simulink model "modelo_asm1_v2"  (R2024a)
settings: Solver=VariableStepAuto  StartTime=0.0  StopTime=28  RelTol=1e-3  AbsTol=Auto  EnableMultiTasking=on
settings Model: Creator=romeroj  LastModifiedBy=ktb21
settings DataIOCC: ExternalInput=dat.data  SaveFormat=Array  SignalLoggingSaveFormat=ModelDataLogs  ReturnWorkspaceOutputs=off
settings OptimizationCC: BooleanDataType=off  ExpressionDepthLimit=2147483647  InitFltsAndDblsToZero=on  LifeSpan=inf
settings DebuggingCC: SaveWithParameterizedLinksMsg=none  UnderspecifiedInitializationDetection=Classic  MergeDetectMultiDrivingBlocksExec=none  SignalResolutionControl=TryResolveAllWithWarning  MultiTaskDSMMsg=warning  MultiTaskCondExecSysMsg=none  FcnCallInpInsideContextMsg=warning  UnconnectedInputMsg=warning  UnconnectedOutputMsg=warning  UnconnectedLineMsg=warning  StateNameClashWarn=warning  SFUnexpectedBacktrackingDiag=warning  SFNoUnconditionalDefaultTransitionDiag=warning  ArithmeticOperatorsInVariantConditions=warning
settings HardwareCC: ProdBitPerPointer=32  ProdBitPerSizeT=32  ProdBitPerPtrDiffT=32  ProdLargestAtomicFloat=None  ProdIntDivRoundTo=Undefined  ProdEndianess=Unspecified  ProdWordSize=32  ProdHWDeviceType=32-bit Generic  TargetUnknown=on
settings ModelReferenceCC: EnableRefExpFcnMdlSchedulingChecks=on  PropagateSignalLabelsOutOfModel=off
settings SFSimCC: SimUseLocalCustomCode=off  SimParseCustomCode=off  CustomCodeUndefinedFunction=UseInterfaceOnly
settings RTWCC: RTWUseLocalCustomCode=off  GPUComputeCapability=3.5
settings CodeAppCC: StateflowObjectComments=on
settings GRTTargetCC: TargetFcnLib=ansi_tfl_tmw.mat  TargetLangStandard=C89/C90 (ANSI)  CombineOutputUpdateFcns=off  GRTInterface=on
settings ConfigComp: CovMetricSettings=dw  CovSaveCumulativeToWorkspaceVar=on  CovSaveSingleToWorkspaceVar=on  CovExternalEMLEnable=off

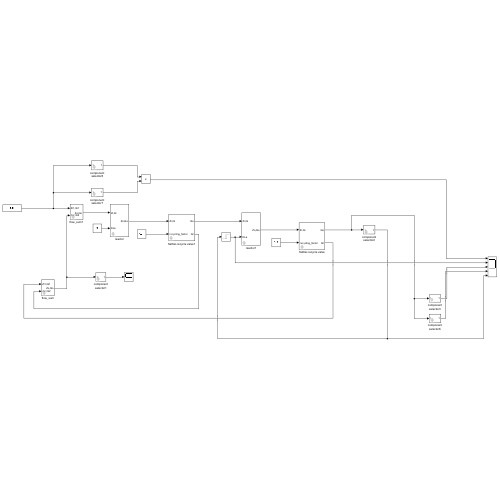
[thumbnail: Simulink's stored preview of the top-level diagram]
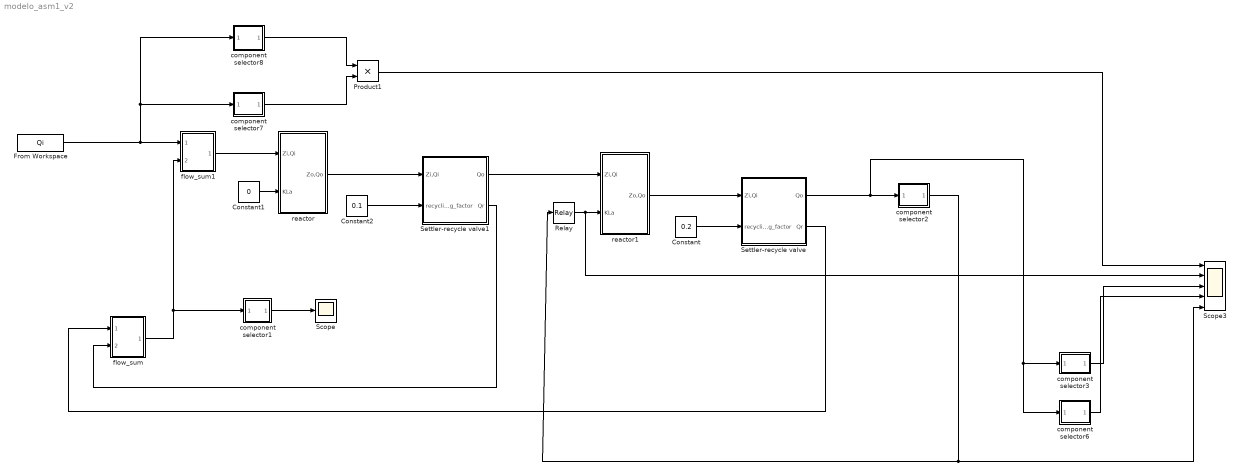
== system modelo_asm1_v2 ==
  Constant : Constant  Value=0.2
  Constant1 : Constant  Value=0
  Constant2 : Constant  Value=0.1
  From Workspace : FromWorkspace  VariableName=Qi  SampleTime=2/1440  ZeroCross=off  OutputAfterFinalValue=Holding final value
  Product1 : Product  RndMeth=Zero
  Relay : Relay  OnSwitchValue=5.4  OffSwitchValue=3  OnOutputValue=40
  Scope : Scope
  Scope3 : Scope  NumInputPorts=5
  Settler-recycle valve : Subsystem  mask{nXi=4, nXs=4, nXbh=4, nXba=4, nXp=4}
      mask prompts: nXi "Xi"; nXs "Xs"; nXbh "Xbh"; nXba "Xba"; nXp "Xp"
      mask DialogControl ParameterTabVar0 Prompt: Settler coefficients
  Settler-recycle valve1 : Subsystem  mask{nXi=0, nXs=0, nXbh=0, nXba=0, nXp=0}
      mask prompts: nXi "Xi"; nXs "Xs"; nXbh "Xbh"; nXba "Xba"; nXp "Xp"
      mask DialogControl ParameterTabVar0 Prompt: Settler coefficients
  component selector1 : Subsystem  mask(Component selection){si=off, ss=off, xi=off, xs=off, xbh=off, xba=off, xp=off, so=off, sno=off, snh=off, snd=off, xnd=off, salk=off, Q=on}
      mask prompts: si "Si: Soluble inert organic matter"; ss "Ss: Readily biodegradable substrate"; xi "Xi: Particulate inert organic matter"; xs "Xs: Slowly biodegradable substrate"; xbh "Xbh: Active heterotrophic biomass"; xba "Xba: Active autotrophic biomass"; xp "Xp: Particulate products arising from biomass decay"; so "So: Oxygen"; sno "Sno: Nitrate and nitrite nitrogen"; snh "Snh: NH 4+ + NH 3 nitrogen"; snd "Snd: Soluble biodegradable organic nitrogen"; xnd "Xnd: Particulate biodegradable organic nitrogen"; salk "Salk: Alkalinity"; Q "Q: Flowrate"
      mask help: Select the components to appear in the output vector of this block.
      mask init:
      | if si
      |     indexx=[1];
      | else
      |     indexx=[];
      | end
      | if ss
      |     indexx=[indexx 2];
      | end
      | if xi
      |     indexx=[indexx 3];
      | end
      | if xs
      |     indexx=[indexx 4];
      | end
      | if xbh
      |     indexx=[indexx 5];
      | end
      | if xba
      |     indexx=[indexx 6];
      | end
      | if xp
      |     indexx=[indexx 7];
      | end
      | if so
      |     indexx=[indexx 8];
      | end
      | if sno
      |     indexx=[indexx 9];
      | end
      | if snh
      |     indexx=[indexx 10];
      | end
      | if snd
      |     indexx=[indexx 11];
      | end
      | if xnd
      |     indexx=[indexx 12];
      | end
      | if salk
      |     indexx=[indexx 13]
      | end
      | if Q
      |     indexx=[indexx 14]
      | end
  component selector2 : Subsystem  mask(Component selection){si=off, ss=off, xi=off, xs=off, xbh=off, xba=off, xp=off, so=off, sno=off, snh=on, snd=off, xnd=off, salk=off, Q=off}
      mask prompts: si "Si: Soluble inert organic matter"; ss "Ss: Readily biodegradable substrate"; xi "Xi: Particulate inert organic matter"; xs "Xs: Slowly biodegradable substrate"; xbh "Xbh: Active heterotrophic biomass"; xba "Xba: Active autotrophic biomass"; xp "Xp: Particulate products arising from biomass decay"; so "So: Oxygen"; sno "Sno: Nitrate and nitrite nitrogen"; snh "Snh: NH 4+ + NH 3 nitrogen"; snd "Snd: Soluble biodegradable organic nitrogen"; xnd "Xnd: Particulate biodegradable organic nitrogen"; salk "Salk: Alkalinity"; Q "Q: Flowrate"
      mask help: Select the components to appear in the output vector of this block.
      mask init: same as modelo_asm1_v2/component selector1
  component selector3 : Subsystem  mask(Component selection){si=off, ss=off, xi=off, xs=off, xbh=off, xba=off, xp=off, so=on, sno=off, snh=off, snd=off, xnd=off, salk=off, Q=off}
      mask prompts: si "Si: Soluble inert organic matter"; ss "Ss: Readily biodegradable substrate"; xi "Xi: Particulate inert organic matter"; xs "Xs: Slowly biodegradable substrate"; xbh "Xbh: Active heterotrophic biomass"; xba "Xba: Active autotrophic biomass"; xp "Xp: Particulate products arising from biomass decay"; so "So: Oxygen"; sno "Sno: Nitrate and nitrite nitrogen"; snh "Snh: NH 4+ + NH 3 nitrogen"; snd "Snd: Soluble biodegradable organic nitrogen"; xnd "Xnd: Particulate biodegradable organic nitrogen"; salk "Salk: Alkalinity"; Q "Q: Flowrate"
      mask help: Select the components to appear in the output vector of this block.
      mask init: same as modelo_asm1_v2/component selector1
  component selector6 : Subsystem  mask(Component selection){si=off, ss=off, xi=on, xs=off, xbh=off, xba=off, xp=off, so=off, sno=off, snh=off, snd=off, xnd=off, salk=off, Q=off}
      mask prompts: si "Si: Soluble inert organic matter"; ss "Ss: Readily biodegradable substrate"; xi "Xi: Particulate inert organic matter"; xs "Xs: Slowly biodegradable substrate"; xbh "Xbh: Active heterotrophic biomass"; xba "Xba: Active autotrophic biomass"; xp "Xp: Particulate products arising from biomass decay"; so "So: Oxygen"; sno "Sno: Nitrate and nitrite nitrogen"; snh "Snh: NH 4+ + NH 3 nitrogen"; snd "Snd: Soluble biodegradable organic nitrogen"; xnd "Xnd: Particulate biodegradable organic nitrogen"; salk "Salk: Alkalinity"; Q "Q: Flowrate"
      mask help: Select the components to appear in the output vector of this block.
      mask init: same as modelo_asm1_v2/component selector1
  component selector7 : Subsystem  mask(Component selection){si=off, ss=off, xi=off, xs=off, xbh=off, xba=off, xp=off, so=off, sno=off, snh=off, snd=off, xnd=off, salk=off, Q=on}
      mask prompts: si "Si: Soluble inert organic matter"; ss "Ss: Readily biodegradable substrate"; xi "Xi: Particulate inert organic matter"; xs "Xs: Slowly biodegradable substrate"; xbh "Xbh: Active heterotrophic biomass"; xba "Xba: Active autotrophic biomass"; xp "Xp: Particulate products arising from biomass decay"; so "So: Oxygen"; sno "Sno: Nitrate and nitrite nitrogen"; snh "Snh: NH 4+ + NH 3 nitrogen"; snd "Snd: Soluble biodegradable organic nitrogen"; xnd "Xnd: Particulate biodegradable organic nitrogen"; salk "Salk: Alkalinity"; Q "Q: Flowrate"
      mask help: Select the components to appear in the output vector of this block.
      mask init: same as modelo_asm1_v2/component selector1
  component selector8 : Subsystem  mask(Component selection){si=off, ss=off, xi=off, xs=off, xbh=off, xba=off, xp=off, so=off, sno=off, snh=on, snd=off, xnd=off, salk=off, Q=off}
      mask prompts: si "Si: Soluble inert organic matter"; ss "Ss: Readily biodegradable substrate"; xi "Xi: Particulate inert organic matter"; xs "Xs: Slowly biodegradable substrate"; xbh "Xbh: Active heterotrophic biomass"; xba "Xba: Active autotrophic biomass"; xp "Xp: Particulate products arising from biomass decay"; so "So: Oxygen"; sno "Sno: Nitrate and nitrite nitrogen"; snh "Snh: NH 4+ + NH 3 nitrogen"; snd "Snd: Soluble biodegradable organic nitrogen"; xnd "Xnd: Particulate biodegradable organic nitrogen"; salk "Salk: Alkalinity"; Q "Q: Flowrate"
      mask help: Select the components to appear in the output vector of this block.
      mask init: same as modelo_asm1_v2/component selector1
  flow_sum : Subsystem
      mask help: Sum two flows
  flow_sum1 : Subsystem
      mask help: Sum two flows
  reactor : Subsystem  mask{Si0=30, Ss0=69.5, Xi0=51.2, Xs0=202.32, Xbh0=28.17, Xba0=25, Xp0=0, So0=0, Sno0=0, Snh0=5, Snd0=6.95, Xnd0=5, Salk0=7, Yh=0.67, Ya=0.24, ixb=0.08, fp=0.08, ixp=0.06, muh=4, Ks=10, Koh=0.2, Kno=0.5, ng=0.8, mua=0.8, Knh=1, Koa=0.4, bh=0.3, ba=0.05, ka=0.05, kh=3, Kx=0.1, nh=0.8, So_sat=10, Vol=5400}
      mask prompts: Si0 "Si: Soluble inert organic matter [g_COD m^-3]"; Ss0 "Ss: Readily biodegradable substrate [g_COD m^-3]"; Xi0 "Xi: Particulate inert organic matter [g_COD m^-3]"; Xs0 "Xs: Slowly biodegradable substrate [g_COD m^-3]"; Xbh0 "Xbh: Active heterotrophic biomass [g_COD m^-3]"; Xba0 "Xba: Active autotrophic biomass [g_COD m^-3]"; Xp0 "Xp: Particulate products arising from biomass decay"; So0 "So: Oxygen [g_O m^-3]"; Sno0 "Sno: Nitrate and nitrite nitrogen [g_N m^-3]"; Snh0 "Snh: NH 4+ + NH 3 nitrogen [g_N m^-3]"; Snd0 "Snd: Soluble biodegradable organic nitrogen [g_N m^-3]"; Xnd0 "Xnd:  Particulate biodegradable organic nitrogen [g_N m^-3]"; Salk0 "Salk: Alkalinity"; Yh "Yh: Yield for heterotrophic biomass"; Ya "Ya: Yield for autotrophic biomass"; ixb "ixb: Mass of biomass per mass of COD in biomass [g_N g_COD^-1 ]"; fp "fp: Fraction of biomass leading to particulate products [-]"; ixp "ixp: Mass of biomass per mass of COD in products from biomass decay [g_N g_COD^-1]"; muh "muh: Maximum specific growth rate for heterotrophic biomass [day^-1]"; Ks "Ks: Half-saturation coefficient for heterotrophic biomass [g_COD m^-3]"; Koh "Koh: Nitrate half-saturation coefficient for denitrifying het- erotrophic biomass [g_N m^-3]"; Kno "Kno: Oxygen half-saturation coefficient for heterotrophic biomass [g_O2 m^-3]"; ng "ng: Correction factor for Î¼ H under anoxic conditions [â€“]"; mua "mua: Maximum specific growth rate for autotrophic biomass [day^-1]"; Knh "Knh: Ammonia half-saturation coefficient for autotrophic biomass [g_N m^-3]"; Koa "Koa: Oxygen half-saturation coefficient for autotrophic biomass [gO2 m^-3]"; bh "bh: Decay rate coefficient for heterotrophic biomass [day^-1]"; ba "ba: Decay rate coefficient for autotrophic biomass [day^-1]"; ka "ka: Ammonification rate [m^3 g^-1_COD day^-1]"; kh "kh: Maximum specific hydrolysis rate [day^-1 ]"; Kx "Kx: Half-saturation coefficient for hydrolysis of slowly biodegradable substrate [â€“]"; nh "nh: Correction factor for hydrolysis under anoxic conditions [â€“]"; So_sat "So_sat: Saturated dissolved oxygen concentration [g_O m^-3]"; Vol "Vol: Volume [m^3]"
      mask help: ASM1 model for activate slugets waste water tractement reactor.
      mask init:
      | initial_cond=[Si0 Ss0 Xi0 Xs0 Xbh0 Xba0 Xp0 So0 Sno0 Snh0 Snd0 Xnd0 Salk0];
      | parameters=[Yh Ya ixb fp ixp muh Ks Koh Kno ng mua Knh Koa bh ba ka kh Kx nh So_sat Vol];
      mask DialogControl ParameterTabVar0 Prompt: Initial conditions
      mask DialogControl ParameterTabVar01 Prompt: Parameters
  reactor1 : Subsystem  mask{Si0=30, Ss0=69.5, Xi0=51.2, Xs0=202.32, Xbh0=28.17, Xba0=25, Xp0=0, So0=0, Sno0=0, Snh0=5, Snd0=6.95, Xnd0=5, Salk0=7, Yh=0.67, Ya=0.24, ixb=0.08, fp=0.08, ixp=0.06, muh=4, Ks=10, Koh=0.2, Kno=0.5, ng=0.8, mua=0.8, Knh=1, Koa=0.4, bh=0.3, ba=0.05, ka=0.05, kh=3, Kx=0.1, nh=0.8, So_sat=10, Vol=5400}
      mask prompts: Si0 "Si: Soluble inert organic matter [g_COD m^-3]"; Ss0 "Ss: Readily biodegradable substrate [g_COD m^-3]"; Xi0 "Xi: Particulate inert organic matter [g_COD m^-3]"; Xs0 "Xs: Slowly biodegradable substrate [g_COD m^-3]"; Xbh0 "Xbh: Active heterotrophic biomass [g_COD m^-3]"; Xba0 "Xba: Active autotrophic biomass [g_COD m^-3]"; Xp0 "Xp: Particulate products arising from biomass decay"; So0 "So: Oxygen [g_O m^-3]"; Sno0 "Sno: Nitrate and nitrite nitrogen [g_N m^-3]"; Snh0 "Snh: NH 4+ + NH 3 nitrogen [g_N m^-3]"; Snd0 "Snd: Soluble biodegradable organic nitrogen [g_N m^-3]"; Xnd0 "Xnd:  Particulate biodegradable organic nitrogen [g_N m^-3]"; Salk0 "Salk: Alkalinity"; Yh "Yh: Yield for heterotrophic biomass"; Ya "Ya: Yield for autotrophic biomass"; ixb "ixb: Mass of biomass per mass of COD in biomass [g_N g_COD^-1 ]"; fp "fp: Fraction of biomass leading to particulate products [-]"; ixp "ixp: Mass of biomass per mass of COD in products from biomass decay [g_N g_COD^-1]"; muh "muh: Maximum specific growth rate for heterotrophic biomass [day^-1]"; Ks "Ks: Half-saturation coefficient for heterotrophic biomass [g_COD m^-3]"; Koh "Koh: Nitrate half-saturation coefficient for denitrifying het- erotrophic biomass [g_N m^-3]"; Kno "Kno: Oxygen half-saturation coefficient for heterotrophic biomass [g_O2 m^-3]"; ng "ng: Correction factor for Î¼ H under anoxic conditions [â€“]"; mua "mua: Maximum specific growth rate for autotrophic biomass [day^-1]"; Knh "Knh: Ammonia half-saturation coefficient for autotrophic biomass [g_N m^-3]"; Koa "Koa: Oxygen half-saturation coefficient for autotrophic biomass [gO2 m^-3]"; bh "bh: Decay rate coefficient for heterotrophic biomass [day^-1]"; ba "ba: Decay rate coefficient for autotrophic biomass [day^-1]"; ka "ka: Ammonification rate [m^3 g^-1_COD day^-1]"; kh "kh: Maximum specific hydrolysis rate [day^-1 ]"; Kx "Kx: Half-saturation coefficient for hydrolysis of slowly biodegradable substrate [â€“]"; nh "nh: Correction factor for hydrolysis under anoxic conditions [â€“]"; So_sat "So_sat: Saturated dissolved oxygen concentration [g_O m^-3]"; Vol "Vol: Volume [m^3]"
      mask help: ASM1 model for activate slugets waste water tractement reactor.
      mask init:
      | initial_cond=[Si0 Ss0 Xi0 Xs0 Xbh0 Xba0 Xp0 So0 Sno0 Snh0 Snd0 Xnd0 Salk0];
      | parameters=[Yh Ya ixb fp ixp muh Ks Koh Kno ng mua Knh Koa bh ba ka kh Kx nh So_sat Vol];
      mask DialogControl ParameterTabVar0 Prompt: Initial conditions
      mask DialogControl ParameterTabVar01 Prompt: Parameters
  wires:
  component selector2/1(Out1) -> Relay/1, Scope3/5
  Constant/1 -> Settler-recycle valve/2(recycling_factor)
  Settler-recycle valve/1(Qo) -> component selector3/1(In1), component selector6/1(In1), component selector2/1(In1)
  component selector3/1(Out1) -> Scope3/3
  component selector8/1(Out1) -> Product1/1
  component selector7/1(Out1) -> Product1/2
  Product1/1 -> Scope3/1
  reactor/1(Zo,Qo) -> Settler-recycle valve1/1(Zi,Qi)
  component selector1/1(Out1) -> Scope/1
  reactor1/1(Zo,Qo) -> Settler-recycle valve/1(Zi,Qi)
  Settler-recycle valve/2(Qr) -> flow_sum/1(Zi1,Qi1)
  Settler-recycle valve1/1(Qo) -> reactor1/1(Zi,Qi)
  flow_sum/1(Zo,Qo) -> flow_sum1/2(Zi2,Qi2), component selector1/1(In1)
  Settler-recycle valve1/2(Qr) -> flow_sum/2(Zi2,Qi2)
  Constant1/1 -> reactor/2(KLa)
  flow_sum1/1(Zo,Qo) -> reactor/1(Zi,Qi)
  Relay/1 -> Scope3/2, reactor1/2(KLa)
  From Workspace/1 -> component selector8/1(In1), component selector7/1(In1), flow_sum1/1(Zi1,Qi1)
  component selector6/1(Out1) -> Scope3/4
  Constant2/1 -> Settler-recycle valve1/2(recycling_factor)

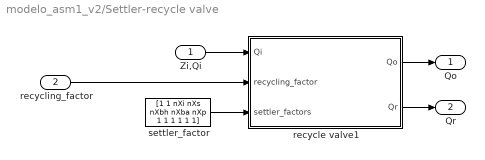
== system modelo_asm1_v2/Settler-recycle valve ==
  Zi,Qi : Inport
  recycling_factor : Inport  Port=2
  recycle valve1 : MATLAB Function  TreatAsAtomicUnit=on
  settler_factor : Constant  Value=[1 1 nXi nXs nXbh nXba nXp 1 1 1 1 1 1]
  Qo : Outport
  Qr : Outport  Port=2
  wires:
  settler_factor/1 -> recycle valve1/3(settler_factors)
  Zi,Qi/1 -> recycle valve1/1(Qi)
  recycling_factor/1 -> recycle valve1/2(recycling_factor)
  recycle valve1/2(Qr) -> Qr/1
  recycle valve1/1(Qo) -> Qo/1

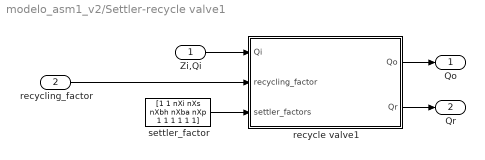
== system modelo_asm1_v2/Settler-recycle valve1 ==
  Zi,Qi : Inport
  recycling_factor : Inport  Port=2
  recycle valve1 : MATLAB Function  TreatAsAtomicUnit=on
  settler_factor : Constant  Value=[1 1 nXi nXs nXbh nXba nXp 1 1 1 1 1 1]
  Qo : Outport
  Qr : Outport  Port=2
  wires:
  recycle valve1/1(Qo) -> Qo/1
  recycle valve1/2(Qr) -> Qr/1
  recycling_factor/1 -> recycle valve1/2(recycling_factor)
  Zi,Qi/1 -> recycle valve1/1(Qi)
  settler_factor/1 -> recycle valve1/3(settler_factors)

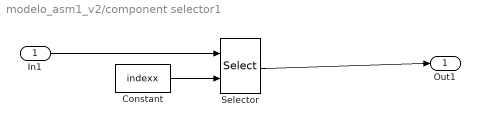
== system modelo_asm1_v2/component selector1 ==
  In1 : Inport
  Constant : Constant  Value=indexx
  Selector : Selector  InputPortWidth=14  IndexOptions=Index vector (port)  Indices=[1 3]  OutputSizes=1
  Out1 : Outport
  wires:
  In1/1 -> Selector/1
  Selector/1 -> Out1/1
  Constant/1 -> Selector/2

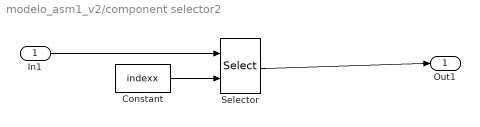
== system modelo_asm1_v2/component selector2 ==
  In1 : Inport
  Constant : Constant  Value=indexx
  Selector : Selector  InputPortWidth=14  IndexOptions=Index vector (port)  Indices=[1 3]  OutputSizes=1
  Out1 : Outport
  wires:
  Constant/1 -> Selector/2
  Selector/1 -> Out1/1
  In1/1 -> Selector/1

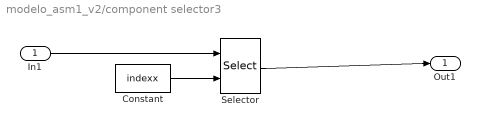
== system modelo_asm1_v2/component selector3 ==
  In1 : Inport
  Constant : Constant  Value=indexx
  Selector : Selector  InputPortWidth=14  IndexOptions=Index vector (port)  Indices=[1 3]  OutputSizes=1
  Out1 : Outport
  wires:
  In1/1 -> Selector/1
  Selector/1 -> Out1/1
  Constant/1 -> Selector/2

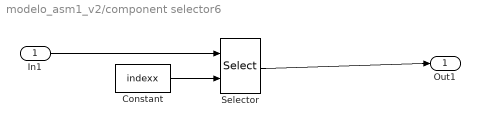
== system modelo_asm1_v2/component selector6 ==
  In1 : Inport
  Constant : Constant  Value=indexx
  Selector : Selector  InputPortWidth=14  IndexOptions=Index vector (port)  Indices=[1 3]  OutputSizes=1
  Out1 : Outport
  wires:
  Constant/1 -> Selector/2
  Selector/1 -> Out1/1
  In1/1 -> Selector/1

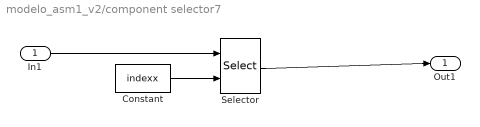
== system modelo_asm1_v2/component selector7 ==
  In1 : Inport
  Constant : Constant  Value=indexx
  Selector : Selector  InputPortWidth=14  IndexOptions=Index vector (port)  Indices=[1 3]  OutputSizes=1
  Out1 : Outport
  wires:
  Constant/1 -> Selector/2
  Selector/1 -> Out1/1
  In1/1 -> Selector/1

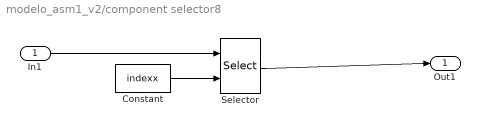
== system modelo_asm1_v2/component selector8 ==
  In1 : Inport
  Constant : Constant  Value=indexx
  Selector : Selector  InputPortWidth=14  IndexOptions=Index vector (port)  Indices=[1 3]  OutputSizes=1
  Out1 : Outport
  wires:
  In1/1 -> Selector/1
  Selector/1 -> Out1/1
  Constant/1 -> Selector/2

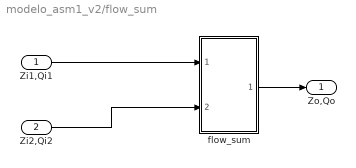
== system modelo_asm1_v2/flow_sum ==
  Zi1,Qi1 : Inport
  Zi2,Qi2 : Inport  Port=2
  flow_sum : Subsystem
      mask DialogControl ParameterTabVar0 Prompt: Settler factors
  Zo,Qo : Outport
  wires:
  Zi2,Qi2/1 -> flow_sum/2(Zi2,Qi2)
  Zi1,Qi1/1 -> flow_sum/1(Zi1,Qi1)
  flow_sum/1(Zo,Qo) -> Zo,Qo/1

== system modelo_asm1_v2/flow_sum1 ==
  Zi1,Qi1 : Inport
  Zi2,Qi2 : Inport  Port=2
  flow_sum : Subsystem
      mask DialogControl ParameterTabVar0 Prompt: Settler factors
  Zo,Qo : Outport
  wires:
  flow_sum/1(Zo,Qo) -> Zo,Qo/1
  Zi1,Qi1/1 -> flow_sum/1(Zi1,Qi1)
  Zi2,Qi2/1 -> flow_sum/2(Zi2,Qi2)

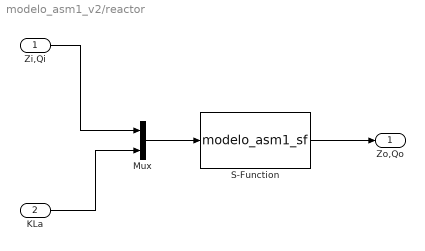
== system modelo_asm1_v2/reactor ==
  Zi,Qi : Inport
  KLa : Inport  Port=2
  Mux : Mux  Inputs=2
  S-Function : S-Function  FunctionName=modelo_asm1_sf  Parameters=initial_cond, parameters  SFunctionDeploymentMode=off  EnableBusSupport=off
  Zo,Qo : Outport
  wires:
  S-Function/1 -> Zo,Qo/1
  Mux/1 -> S-Function/1
  Zi,Qi/1 -> Mux/1
  KLa/1 -> Mux/2

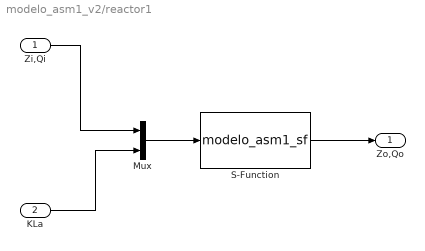
== system modelo_asm1_v2/reactor1 ==
  Zi,Qi : Inport
  KLa : Inport  Port=2
  Mux : Mux  Inputs=2
  S-Function : S-Function  FunctionName=modelo_asm1_sf  Parameters=initial_cond, parameters  SFunctionDeploymentMode=off  EnableBusSupport=off
  Zo,Qo : Outport
  wires:
  KLa/1 -> Mux/2
  Zi,Qi/1 -> Mux/1
  Mux/1 -> S-Function/1
  S-Function/1 -> Zo,Qo/1

== system modelo_asm1_v2/flow_sum/flow_sum ==
  Zi1,Qi1 : Inport
  Zi2,Qi2 : Inport  Port=2
  flow_sum : MATLAB Function  TreatAsAtomicUnit=on
  Zo,Qo : Outport
  wires:
  flow_sum/1(ZoQo) -> Zo,Qo/1
  Zi2,Qi2/1 -> flow_sum/2(Zi2Qi2)
  Zi1,Qi1/1 -> flow_sum/1(Zi1Qi1)

== system modelo_asm1_v2/flow_sum1/flow_sum ==
  Zi1,Qi1 : Inport
  Zi2,Qi2 : Inport  Port=2
  flow_sum : MATLAB Function  TreatAsAtomicUnit=on
  Zo,Qo : Outport
  wires:
  Zi1,Qi1/1 -> flow_sum/1(Zi1Qi1)
  Zi2,Qi2/1 -> flow_sum/2(Zi2Qi2)
  flow_sum/1(ZoQo) -> Zo,Qo/1

== matlab function modelo_asm1_v2/Settler-recycle valve/recycle valve1 ==
  data: Qo output; Qr output; Qi input; recycling_factor input; settler_factors input
function [Qo,Qr]  = fcn(Qi,recycling_factor,settler_factors)
%This block simulates the effect of the settler in the recycle flow.
%Input paramenters:
% -Qi: Input flow
% -sludge_re_conc: concetration of the sludge produced by the settler.
%       The sludge concnetration in the output flows (Qo and Qr) is "sludge_re_conc" times the 
%       the sludge concentration in the input flow (Qi).
% -recycle: percentage of Qi assignet to the output Qr.
%Output paramenters:
% -Qr=recycling_factor*Qi
% -Qo=(1-recycling_factor)*Qi


%#eml


Xi=Qi(1:13);

Xr=settler_factors.*Xi;

Xo=(1-settler_factors*recycling_factor)/(1-recycling_factor).*Xi;

Qr=[Xr; recycling_factor*Qi(end)];

Qo=[Xo; (1-recycling_factor)*Qi(end)];

== matlab function modelo_asm1_v2/flow_sum/flow_sum/flow_sum ==
  data: ZoQo output; Zi1Qi1 input; Zi2Qi2 input
function ZoQo   = fcn(Zi1Qi1,Zi2Qi2)
%This block simulates the the summation of two flows.
%Input paramenters:
% -Qi1 and Qi2: Input flows to be added 
% %Output paramenters:
% -ZoQo: resultan flow 
%#eml

ZoQo=zeros(14,1);
ZoQo(end)=Zi1Qi1(end)+Zi2Qi2(end);
ZoQo(1:end-1)=(Zi1Qi1(1:end-1)*Zi1Qi1(end) + Zi2Qi2(1:end-1)*Zi2Qi2(end))/(Zi1Qi1(end) + Zi2Qi2(end)  +  1e-4);

== matlab function modelo_asm1_v2/Settler-recycle valve1/recycle valve1 ==
  data: Qo output; Qr output; Qi input; recycling_factor input; settler_factors input
function [Qo,Qr]  = fcn(Qi,recycling_factor,settler_factors)
%This block simulates the effect of the settler in the recycle flow.
%Input paramenters:
% -Qi: Input flow
% -sludge_re_conc: concetration of the sludge produced by the settler.
%       The sludge concnetration in the output flows (Qo and Qr) is "sludge_re_conc" times the 
%       the sludge concentration in the input flow (Qi).
% -recycle: percentage of Qi assignet to the output Qr.
%Output paramenters:
% -Qr=recycling_factor*Qi
% -Qo=(1-recycling_factor)*Qi


%#eml


Xi=Qi(1:13);

Xr=settler_factors.*Xi;

Xo=(1-settler_factors*recycling_factor)/(1-recycling_factor).*Xi;

Qr=[Xr; recycling_factor*Qi(end)];

Qo=[Xo; (1-recycling_factor)*Qi(end)];

== matlab function modelo_asm1_v2/flow_sum1/flow_sum/flow_sum ==
  data: ZoQo output; Zi1Qi1 input; Zi2Qi2 input
function ZoQo   = fcn(Zi1Qi1,Zi2Qi2)
%This block simulates the the summation of two flows.
%Input paramenters:
% -Qi1 and Qi2: Input flows to be added 
% %Output paramenters:
% -ZoQo: resultan flow 
%#eml

ZoQo=zeros(14,1);
ZoQo(end)=Zi1Qi1(end)+Zi2Qi2(end);
ZoQo(1:end-1)=(Zi1Qi1(1:end-1)*Zi1Qi1(end) + Zi2Qi2(1:end-1)*Zi2Qi2(end))/(Zi1Qi1(end) + Zi2Qi2(end)  +  1e-4);
